simulink model "SevenInput_Simulink"  (R2022b)
settings: Solver=VariableStepAuto  StartTime=0.0  StopTime=10.0  RelTol=1e-3
settings Model: Creator=yeyi5  LastModifiedBy=yeyi5

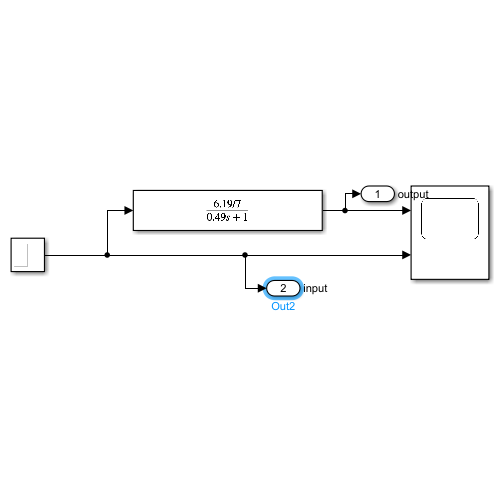
[thumbnail: Simulink's stored preview of the top-level diagram]
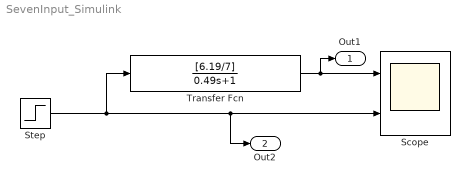
== system SevenInput_Simulink ==
  Scope : Scope  NumInputPorts=2
  Step : Step  After=7  SampleTime=0
  Transfer Fcn : TransferFcn  Numerator=[6.19/7]  Denominator=[0.49 1]
  Out1 : Outport  SignalName=output
  Out2 : Outport  Port=2  SignalName=input
  wires:
  Step/1 -> Transfer Fcn/1, Out2/1, Scope/2
  Transfer Fcn/1 -> Out1/1, Scope/1
